simulink model "dimensions_equivalent"  (R2021b)
settings: Solver=VariableStepAuto  StartTime=0.0  StopTime=10.0  RelTol=1e-3
undefined symbols (not defined in the file): DiscIntNeverNeededParam, magnitude, Newton, Raphson
libraries: simulink x80, slpidlib x2
(part 2 of 3)

== system dimensions_equivalent/tsmc_Slforge53 ==
  tsmc_Slforge1 : Inport
  tsmc_Slforge10 : Delay  SampleTime=1
  tsmc_Slforge3 : DiscreteFilter  SampleTime=1
  tsmc_Slforge4 : Sum  Inputs=+-
  tsmc_Slforge5 : Rounding
  tsmc_Slforge6 : ComplexToRealImag
  tsmc_Slforge7 : Product  Inputs=*
  tsmc_Slforge8 : Polyval  Coefs=[ +2.081618890e-019, -1.441693666e-014, +4.719686976e-010, -8.536869453e-006, +1.621573104e-001, -8.087801117e+001 ]
  tsmc_Slforge9 : Delay  SampleTime=1
  tsmc_Slforge2 : Outport  VectorParamsAs1DForOutWhenUnconnected=off
  wires:
  tsmc_Slforge1/1 -> tsmc_Slforge7/1
  tsmc_Slforge7/1 -> tsmc_Slforge3/1
  tsmc_Slforge4/1 -> tsmc_Slforge8/1
  tsmc_Slforge8/1 -> tsmc_Slforge6/1
  tsmc_Slforge6/1 -> tsmc_Slforge5/1
  tsmc_Slforge3/1 -> tsmc_Slforge2/1
  tsmc_Slforge5/1 -> tsmc_Slforge9/1
  tsmc_Slforge9/1 -> tsmc_Slforge4/2
  tsmc_Slforge6/2 -> tsmc_Slforge10/1
  tsmc_Slforge10/1 -> tsmc_Slforge4/1

== system dimensions_equivalent/tsmc_Slforge54 ==
  tsmc_Slforge1 : Inport
  tsmc_Slforge10 : Inport  Port=2
  tsmc_Slforge11 : Inport  Port=3
  tsmc_Slforge3 : Delay  SampleTime=1
  tsmc_Slforge4 : Polyval  Coefs=[ +2.081618890e-019, -1.441693666e-014, +4.719686976e-010, -8.536869453e-006, +1.621573104e-001, -8.087801117e+001 ]
  tsmc_Slforge5 : Sum  Inputs=+-
  tsmc_Slforge6 : Signum
  tsmc_Slforge7 : Product
  tsmc_Slforge8 : Product  Inputs=*
  tsmc_Slforge9 : Constant  Value=[57292007.464946]  SampleTime=1
  tsmc_Slforge2 : Outport  VectorParamsAs1DForOutWhenUnconnected=off
  wires:
  tsmc_Slforge5/1 -> tsmc_Slforge7/1
  tsmc_Slforge9/1 -> tsmc_Slforge4/1
  tsmc_Slforge10/1 -> tsmc_Slforge3/1
  tsmc_Slforge6/1 -> tsmc_Slforge5/1
  tsmc_Slforge3/1 -> tsmc_Slforge2/1
  tsmc_Slforge4/1 -> tsmc_Slforge8/1
  tsmc_Slforge8/1 -> tsmc_Slforge5/2
  tsmc_Slforge1/1 -> tsmc_Slforge7/2
  tsmc_Slforge11/1 -> tsmc_Slforge6/1

== system dimensions_equivalent/tsmc_Slforge55 ==
  tsmc_Slforge1 : Inport
  tsmc_Slforge3 : simulink/Discrete/Transfer Fcn First Order  PoleZ=0.95  ICPrevOutput=0.0  DoSatur=off
  tsmc_Slforge4 : Math  Operator=log10  SignedPower=on  SaturateOnIntegerOverflow=on
  tsmc_Slforge5 : Product
  tsmc_Slforge6 : Product  Inputs=**
  tsmc_Slforge7 : Rounding
  tsmc_Slforge8 : Delay  SampleTime=1
  tsmc_Slforge9 : Delay  SampleTime=1
  tsmc_Slforge2 : Outport  VectorParamsAs1DForOutWhenUnconnected=off
  wires:
  tsmc_Slforge6/1 -> tsmc_Slforge4/1
  tsmc_Slforge7/1 -> tsmc_Slforge2/1, tsmc_Slforge9/1
  tsmc_Slforge1/1 -> tsmc_Slforge6/1
  tsmc_Slforge3/1 -> tsmc_Slforge7/1, tsmc_Slforge5/2
  tsmc_Slforge4/1 -> tsmc_Slforge5/1
  tsmc_Slforge5/1 -> tsmc_Slforge8/1
  tsmc_Slforge8/1 -> tsmc_Slforge6/2
  tsmc_Slforge9/1 -> tsmc_Slforge3/1

== system dimensions_equivalent/tsmc_Slforge56 ==
  tsmc_Slforge1 : Inport
  tsmc_Slforge10 : Delay  SampleTime=1
  tsmc_Slforge3 : DiscreteFir  SampleTime=1
  tsmc_Slforge4 : Rounding
  tsmc_Slforge5 : Reshape
  tsmc_Slforge6 : Bias  Bias=[938444470.111902]
  tsmc_Slforge7 : Squeeze
  tsmc_Slforge8 : Trigonometry
  tsmc_Slforge9 : Delay  SampleTime=1
  tsmc_Slforge2 : Outport  VectorParamsAs1DForOutWhenUnconnected=off
  wires:
  tsmc_Slforge4/1 -> tsmc_Slforge6/1
  tsmc_Slforge6/1 -> tsmc_Slforge2/1
  tsmc_Slforge5/1 -> tsmc_Slforge7/1
  tsmc_Slforge3/1 -> tsmc_Slforge8/1
  tsmc_Slforge1/1 -> tsmc_Slforge4/1
  tsmc_Slforge8/1 -> tsmc_Slforge9/1
  tsmc_Slforge9/1 -> tsmc_Slforge3/1
  tsmc_Slforge7/1 -> tsmc_Slforge10/1
  tsmc_Slforge10/1 -> tsmc_Slforge5/1

== system dimensions_equivalent/tsmc_Slforge74 ==
  tsmc_Slforge1 : Inport
  tsmc_Slforge23 : Inport  Port=2
  tsmc_Slforge24 : Inport  Port=3
  tsmc_Slforge25 : Inport  Port=4
  Action Port : ActionPort  ActionPortLabel=if { }
  tsmc_Slforge10 : MinMax  Function=max  Inputs=2
  tsmc_Slforge11 : Gain  Gain=[-950435742.515709]
  tsmc_Slforge12 : Sin  TimeSource=Use external signal  SampleTime=0
  tsmc_Slforge13 : Product  Inputs=*
  tsmc_Slforge14 : MinMax  Inputs=3
  tsmc_Slforge15 : Squeeze
  tsmc_Slforge16 : Sum  Inputs=+
  tsmc_Slforge17 : Polyval  Coefs=[ +2.081618890e-019, -1.441693666e-014, +4.719686976e-010, -8.536869453e-006, +1.621573104e-001, -8.087801117e+001 ]
  tsmc_Slforge18 : DotProduct  InputSameDT=on  OutDataTypeStr=Inherit: Inherit via internal rule
  tsmc_Slforge19 : Sin  TimeSource=Use external signal  SampleTime=0
  tsmc_Slforge20 : Sum  Inputs=-+
  tsmc_Slforge21 : Constant  Value=[772260001.144114]  SampleTime=1
  tsmc_Slforge22 : Constant  Value=[-948406195.487638]  SampleTime=1
  tsmc_Slforge26 : Delay
  tsmc_Slforge27 : Delay
  tsmc_Slforge3 : simulink/Discrete/Transfer Fcn Real Zero  ZeroZ=0.75  ICPrevInput=0.0  DoSatur=off
      settings: SourceProductBaseCode=SL
  tsmc_Slforge4 : simulink/Discrete/Transfer Fcn Lead or Lag  PoleZ=0.95  ZeroZ=0.75  ICPrevOutput=0.0  ICPrevInput=0.0  DoSatur=off
      settings: SourceProductBaseCode=SL
  tsmc_Slforge5 : Sum  Inputs=+-
  tsmc_Slforge6 : simulink/Math Operations/Slider Gain  gain=1  low=0  high=2
  tsmc_Slforge7 : Sqrt  Operator=rSqrt  AlgorithmType=Newton-Raphson  SaturateOnIntegerOverflow=on
  tsmc_Slforge8 : Product
  tsmc_Slforge9 : Sum
  tsmc_Slforge2 : Outport  VectorParamsAs1DForOutWhenUnconnected=off
  wires:
  tsmc_Slforge16/1 -> tsmc_Slforge15/1
  tsmc_Slforge23/1 -> tsmc_Slforge3/1, tsmc_Slforge19/1
  tsmc_Slforge25/1 -> tsmc_Slforge17/1
  tsmc_Slforge21/1 -> tsmc_Slforge20/1
  tsmc_Slforge4/1 -> tsmc_Slforge7/1
  tsmc_Slforge20/1 -> tsmc_Slforge2/1
  tsmc_Slforge6/1 -> tsmc_Slforge18/1
  tsmc_Slforge3/1 -> tsmc_Slforge5/2
  tsmc_Slforge18/1 -> tsmc_Slforge9/1
  tsmc_Slforge17/1 -> tsmc_Slforge10/1
  tsmc_Slforge12/1 -> tsmc_Slforge11/1
  tsmc_Slforge13/1 -> tsmc_Slforge8/1
  tsmc_Slforge8/1 -> tsmc_Slforge20/2
  tsmc_Slforge14/1 -> tsmc_Slforge6/1
  tsmc_Slforge22/1 -> tsmc_Slforge18/2, tsmc_Slforge4/1
  tsmc_Slforge24/1 -> tsmc_Slforge13/1
  tsmc_Slforge9/1 -> tsmc_Slforge10/2
  tsmc_Slforge15/1 -> tsmc_Slforge14/2
  tsmc_Slforge1/1 -> tsmc_Slforge8/2
  tsmc_Slforge5/1 -> tsmc_Slforge12/1
  tsmc_Slforge19/1 -> tsmc_Slforge16/1, tsmc_Slforge9/2
  tsmc_Slforge7/1 -> tsmc_Slforge14/3
  tsmc_Slforge11/1 -> tsmc_Slforge26/1
  tsmc_Slforge26/1 -> tsmc_Slforge5/1
  tsmc_Slforge10/1 -> tsmc_Slforge27/1
  tsmc_Slforge27/1 -> tsmc_Slforge14/1

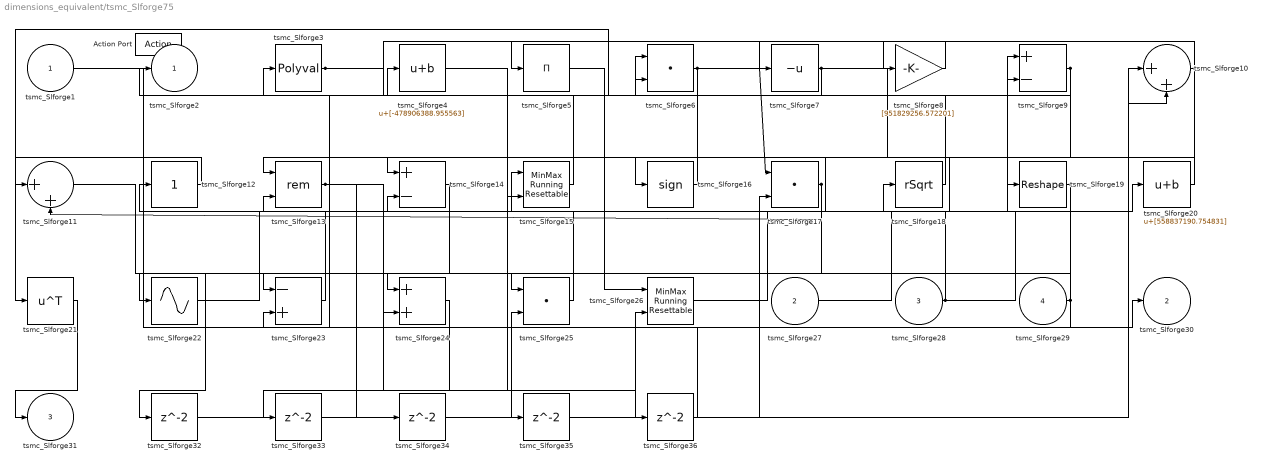
== system dimensions_equivalent/tsmc_Slforge75 ==
  tsmc_Slforge1 : Inport
  tsmc_Slforge27 : Inport  Port=2
  tsmc_Slforge28 : Inport  Port=3
  tsmc_Slforge29 : Inport  Port=4
  Action Port : ActionPort  ActionPortLabel=else { }
  tsmc_Slforge10 : Sum  Inputs=|++
  tsmc_Slforge11 : Sum  Inputs=|++
  tsmc_Slforge12 : simulink/Math Operations/Slider Gain  gain=1  low=0  high=2
  tsmc_Slforge13 : Math  Operator=rem  SignedPower=on  SaturateOnIntegerOverflow=on
  tsmc_Slforge14 : Sum  Inputs=+-
  tsmc_Slforge15 : simulink/Math Operations/MinMax Running Resettable  Function=min  vinit=0.0
  tsmc_Slforge16 : Signum
  tsmc_Slforge17 : DotProduct  InputSameDT=on  OutDataTypeStr=Inherit: Inherit via internal rule
  tsmc_Slforge18 : Sqrt  Operator=rSqrt  AlgorithmType=Newton-Raphson  SaturateOnIntegerOverflow=on
  tsmc_Slforge19 : Reshape
  tsmc_Slforge20 : Bias  Bias=[558837190.754831]
  tsmc_Slforge21 : Math  Operator=transpose  SignedPower=on  SaturateOnIntegerOverflow=on
  tsmc_Slforge22 : Sin  TimeSource=Use external signal  SampleTime=0
  tsmc_Slforge23 : Sum  Inputs=-+
  tsmc_Slforge24 : Sum
  tsmc_Slforge25 : DotProduct  InputSameDT=on  OutDataTypeStr=Inherit: Inherit via internal rule
  tsmc_Slforge26 : simulink/Math Operations/MinMax Running Resettable  Function=min  vinit=0.0
  tsmc_Slforge3 : Polyval  Coefs=[ +2.081618890e-019, -1.441693666e-014, +4.719686976e-010, -8.536869453e-006, +1.621573104e-001, -8.087801117e+001 ]
  tsmc_Slforge{32..36} (5 alike) : Delay
  tsmc_Slforge4 : Bias  Bias=[-478906388.955563]
  tsmc_Slforge5 : Product  Inputs=*
  tsmc_Slforge6 : DotProduct  InputSameDT=on  OutDataTypeStr=Inherit: Inherit via internal rule
  tsmc_Slforge7 : UnaryMinus
  tsmc_Slforge8 : Gain  Gain=[951829256.572201]
  tsmc_Slforge9 : Sum  Inputs=+-
  tsmc_Slforge2 : Outport  VectorParamsAs1DForOutWhenUnconnected=off
  tsmc_Slforge30 : Outport  Port=2  VectorParamsAs1DForOutWhenUnconnected=off
  tsmc_Slforge31 : Outport  Port=3  VectorParamsAs1DForOutWhenUnconnected=off
  wires:
  tsmc_Slforge28/1 -> tsmc_Slforge20/1, tsmc_Slforge15/1
  tsmc_Slforge1/1 -> tsmc_Slforge30/1
  tsmc_Slforge5/1 -> tsmc_Slforge26/1
  tsmc_Slforge18/1 -> tsmc_Slforge21/1
  tsmc_Slforge17/1 -> tsmc_Slforge25/1, tsmc_Slforge11/2
  tsmc_Slforge9/1 -> tsmc_Slforge16/1, tsmc_Slforge2/1
  tsmc_Slforge15/1 -> tsmc_Slforge4/1
  tsmc_Slforge19/1 -> tsmc_Slforge24/1, tsmc_Slforge24/2
  tsmc_Slforge25/1 -> tsmc_Slforge12/1
  tsmc_Slforge11/1 -> tsmc_Slforge23/1
  tsmc_Slforge10/1 -> tsmc_Slforge14/1, tsmc_Slforge7/1
  tsmc_Slforge8/1 -> tsmc_Slforge5/1
  tsmc_Slforge16/1 -> tsmc_Slforge6/1
  tsmc_Slforge21/1 -> tsmc_Slforge31/1
  tsmc_Slforge29/1 -> tsmc_Slforge18/1, tsmc_Slforge22/1, tsmc_Slforge23/2
  tsmc_Slforge22/1 -> tsmc_Slforge14/2
  tsmc_Slforge12/1 -> tsmc_Slforge11/1
  tsmc_Slforge20/1 -> tsmc_Slforge13/1
  tsmc_Slforge6/1 -> tsmc_Slforge17/1, tsmc_Slforge15/2
  tsmc_Slforge23/1 -> tsmc_Slforge13/2
  tsmc_Slforge26/1 -> tsmc_Slforge10/2
  tsmc_Slforge27/1 -> tsmc_Slforge9/1
  tsmc_Slforge7/1 -> tsmc_Slforge19/1, tsmc_Slforge6/2
  tsmc_Slforge3/1 -> tsmc_Slforge8/1, tsmc_Slforge9/2
  tsmc_Slforge13/1 -> tsmc_Slforge34/1, tsmc_Slforge35/1
  tsmc_Slforge14/1 -> tsmc_Slforge32/1
  tsmc_Slforge32/1 -> tsmc_Slforge26/2
  tsmc_Slforge24/1 -> tsmc_Slforge33/1
  tsmc_Slforge33/1 -> tsmc_Slforge10/1
  tsmc_Slforge34/1 -> tsmc_Slforge25/2
  tsmc_Slforge35/1 -> tsmc_Slforge17/2
  tsmc_Slforge4/1 -> tsmc_Slforge36/1
  tsmc_Slforge36/1 -> tsmc_Slforge3/1

== system dimensions_equivalent/tsmc_Slforge76 ==
  tsmc_Slforge1 : Inport
  tsmc_Slforge23 : Inport  Port=2
  Action Port : ActionPort  ActionPortLabel=if { }
  tsmc_Slforge10 : PermuteDimensions
  tsmc_Slforge11 : simulink/Math Operations/Slider Gain  gain=1  low=0  high=2
  tsmc_Slforge12 : Product  Inputs=*
  tsmc_Slforge13 : Assignment  DiagnosticForDimensions=Warning  IndexOptions=Index vector (dialog)  Indices=1  OutputSizes=1
  tsmc_Slforge14 : Sum  Inputs=+-
  tsmc_Slforge15 : Sqrt  SaturateOnIntegerOverflow=on
  tsmc_Slforge16 : MinMax  Function=max  Inputs=3
  tsmc_Slforge17 : Trigonometry
  tsmc_Slforge18 : simulink/Math Operations/Slider Gain  gain=1  low=0  high=2
  tsmc_Slforge19 : Sum  Inputs=+
  tsmc_Slforge20 : Bias  Bias=[872641712.418496]
  tsmc_Slforge21 : Constant  Value=[-855607815.894000]  SampleTime=1
  tsmc_Slforge22 : Constant  Value=[-549961710.513613]  SampleTime=1
  tsmc_Slforge{3,25..28} (5 alike) : Delay
  tsmc_Slforge4 : simulink/Discrete/Tapped Delay  vinit=0.0  samptime=-1  NumDelays=1  DelayOrder=Oldest  includeCurrent=off
  tsmc_Slforge5 : Delay  DelayLengthSource=Input port
      settings: InputPortMap=u0,p1
  tsmc_Slforge6 : Sum  Inputs=--
  tsmc_Slforge7 : Sqrt  SaturateOnIntegerOverflow=on
  tsmc_Slforge8 : Sum  Inputs=--
  tsmc_Slforge9 : Sin  TimeSource=Use external signal  SampleTime=0
  tsmc_Slforge2 : Outport  VectorParamsAs1DForOutWhenUnconnected=off
  tsmc_Slforge24 : Outport  Port=2  VectorParamsAs1DForOutWhenUnconnected=off
  wires:
  tsmc_Slforge8/1 -> tsmc_Slforge16/1, tsmc_Slforge13/2
  tsmc_Slforge4/1 -> tsmc_Slforge5/1
  tsmc_Slforge12/1 -> tsmc_Slforge6/1
  tsmc_Slforge6/1 -> tsmc_Slforge10/1
  tsmc_Slforge5/1 -> tsmc_Slforge18/1
  tsmc_Slforge14/1 -> tsmc_Slforge9/1
  tsmc_Slforge22/1 -> tsmc_Slforge13/1
  tsmc_Slforge18/1 -> tsmc_Slforge11/1, tsmc_Slforge2/1
  tsmc_Slforge3/1 -> tsmc_Slforge15/1
  tsmc_Slforge16/1 -> tsmc_Slforge24/1
  tsmc_Slforge19/1 -> tsmc_Slforge12/1
  tsmc_Slforge13/1 -> tsmc_Slforge17/1
  tsmc_Slforge9/1 -> tsmc_Slforge8/1, tsmc_Slforge16/3
  tsmc_Slforge21/1 -> tsmc_Slforge19/1
  tsmc_Slforge10/1 -> tsmc_Slforge7/1, tsmc_Slforge20/1, tsmc_Slforge8/2
  tsmc_Slforge1/1 -> tsmc_Slforge14/2
  tsmc_Slforge11/1 -> tsmc_Slforge6/2
  tsmc_Slforge23/1 -> tsmc_Slforge16/2
  tsmc_Slforge17/1 -> tsmc_Slforge25/1
  tsmc_Slforge25/1 -> tsmc_Slforge14/1
  tsmc_Slforge15/1 -> tsmc_Slforge26/1
  tsmc_Slforge26/1 -> tsmc_Slforge3/1
  tsmc_Slforge7/1 -> tsmc_Slforge27/1
  tsmc_Slforge27/1 -> tsmc_Slforge4/1
  tsmc_Slforge20/1 -> tsmc_Slforge28/1
  tsmc_Slforge28/1 -> tsmc_Slforge5/2

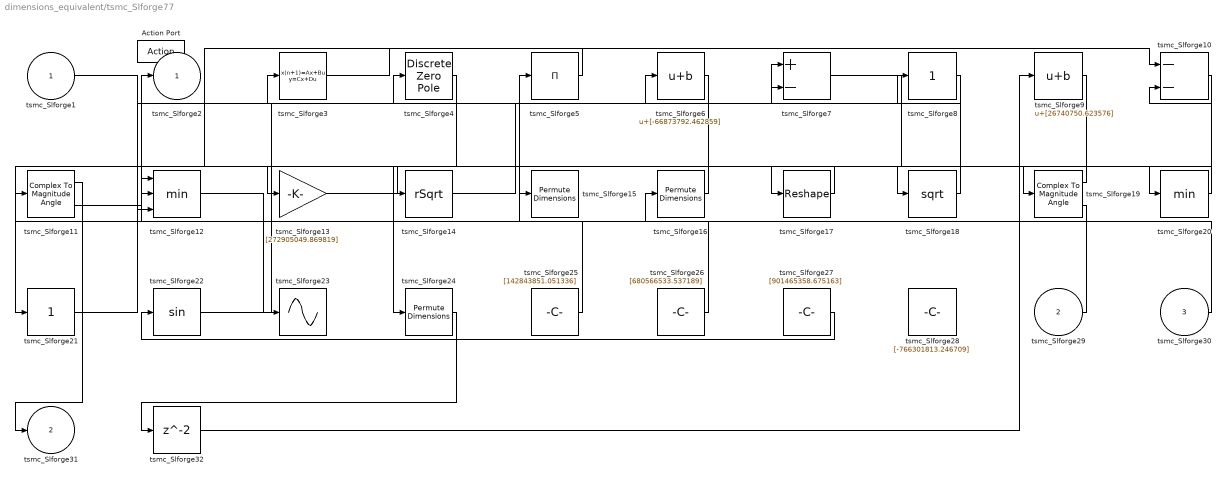
== system dimensions_equivalent/tsmc_Slforge77 ==
  tsmc_Slforge1 : Inport
  tsmc_Slforge29 : Inport  Port=2
  tsmc_Slforge30 : Inport  Port=3
  Action Port : ActionPort  ActionPortLabel=else { }
  tsmc_Slforge10 : Sum  Inputs=--
  tsmc_Slforge11 : ComplexToMagnitudeAngle
  tsmc_Slforge12 : MinMax  Inputs=3
  tsmc_Slforge13 : Gain  Gain=[272905049.869819]
  tsmc_Slforge14 : Sqrt  Operator=rSqrt  AlgorithmType=Newton-Raphson  SaturateOnIntegerOverflow=on
  tsmc_Slforge15 : PermuteDimensions
  tsmc_Slforge16 : PermuteDimensions
  tsmc_Slforge17 : Reshape
  tsmc_Slforge18 : Sqrt  SaturateOnIntegerOverflow=on
  tsmc_Slforge19 : ComplexToMagnitudeAngle
  tsmc_Slforge20 : MinMax
  tsmc_Slforge21 : simulink/Math Operations/Slider Gain  gain=1  low=0  high=2
  tsmc_Slforge22 : Trigonometry
  tsmc_Slforge23 : Sin  TimeSource=Use external signal  SampleTime=0
  tsmc_Slforge24 : PermuteDimensions
  tsmc_Slforge25 : Constant  Value=[142843851.051336]  SampleTime=1
  tsmc_Slforge26 : Constant  Value=[680566533.537189]  SampleTime=1
  tsmc_Slforge27 : Constant  Value=[901465358.675163]  SampleTime=1
  tsmc_Slforge28 : Constant  Value=[-766301813.246709]  SampleTime=1
  tsmc_Slforge3 : DiscreteStateSpace  SampleTime=-1
  tsmc_Slforge32 : Delay
  tsmc_Slforge4 : DiscreteZeroPole  Poles=[0 0.5]  Gain=1  SampleTime=-1
  tsmc_Slforge5 : Product  Inputs=*
  tsmc_Slforge6 : Bias  Bias=[-66873792.462859]
  tsmc_Slforge7 : Sum  Inputs=+-
  tsmc_Slforge8 : simulink/Math Operations/Slider Gain  gain=1  low=0  high=2
  tsmc_Slforge9 : Bias  Bias=[26740750.623576]
  tsmc_Slforge2 : Outport  VectorParamsAs1DForOutWhenUnconnected=off
  tsmc_Slforge31 : Outport  Port=2  VectorParamsAs1DForOutWhenUnconnected=off
  wires:
  tsmc_Slforge30/1 -> tsmc_Slforge5/1
  tsmc_Slforge5/1 -> tsmc_Slforge21/1
  tsmc_Slforge22/1 -> tsmc_Slforge4/1
  tsmc_Slforge13/1 -> tsmc_Slforge20/1
  tsmc_Slforge17/1 -> tsmc_Slforge15/1
  tsmc_Slforge9/1 -> tsmc_Slforge24/1
  tsmc_Slforge27/1 -> tsmc_Slforge22/1
  tsmc_Slforge18/1 -> tsmc_Slforge7/1
  tsmc_Slforge4/1 -> tsmc_Slforge13/1
  tsmc_Slforge25/1 -> tsmc_Slforge11/1
  tsmc_Slforge14/1 -> tsmc_Slforge7/2
  tsmc_Slforge16/1 -> tsmc_Slforge6/1
  tsmc_Slforge21/1 -> tsmc_Slforge3/1
  tsmc_Slforge8/1 -> tsmc_Slforge18/1
  tsmc_Slforge3/1 -> tsmc_Slforge10/1
  tsmc_Slforge29/1 -> tsmc_Slforge14/1
  tsmc_Slforge26/1 -> tsmc_Slforge2/1
  tsmc_Slforge19/1 -> tsmc_Slforge17/1
  tsmc_Slforge20/1 -> tsmc_Slforge10/2
  tsmc_Slforge6/1 -> tsmc_Slforge12/1
  tsmc_Slforge11/1 -> tsmc_Slforge31/1
  tsmc_Slforge19/2 -> tsmc_Slforge16/1
  tsmc_Slforge12/1 -> tsmc_Slforge23/1
  tsmc_Slforge11/2 -> tsmc_Slforge12/2
  tsmc_Slforge7/1 -> tsmc_Slforge19/1
  tsmc_Slforge1/1 -> tsmc_Slforge8/1
  tsmc_Slforge10/1 -> tsmc_Slforge12/3
  tsmc_Slforge24/1 -> tsmc_Slforge32/1
  tsmc_Slforge32/1 -> tsmc_Slforge9/1

== system dimensions_equivalent/tsmc_Slforge78 ==
  tsmc_Slforge1 : Inport
  tsmc_Slforge20 : Inport  Port=2
  tsmc_Slforge21 : Inport  Port=3
  tsmc_Slforge22 : Inport  Port=4
  tsmc_Slforge23 : Inport  Port=5
  tsmc_Slforge24 : Inport  Port=6
  Action Port : ActionPort  ActionPortLabel=if { }
  tsmc_Slforge10 : MinMax  Function=max  Inputs=2
  tsmc_Slforge11 : Reshape
  tsmc_Slforge12 : Bias  Bias=[772438842.352747]
  tsmc_Slforge13 : Polyval  Coefs=[ +2.081618890e-019, -1.441693666e-014, +4.719686976e-010, -8.536869453e-006, +1.621573104e-001, -8.087801117e+001 ]
  tsmc_Slforge14 : Squeeze
  tsmc_Slforge15 : MinMax  Function=max
  tsmc_Slforge16 : MinMax  Function=max  Inputs=3
  tsmc_Slforge17 : Constant  Value=[-48406649.687781]  SampleTime=1
  tsmc_Slforge18 : Constant  Value=[-479832900.428704]  SampleTime=1
  tsmc_Slforge19 : Constant  Value=[314816186.317253]  SampleTime=1
  tsmc_Slforge3 : simulink/Discrete/Difference  ICPrevInput=0.0  OutMin=[]  OutMax=[]  OutDataTypeStr=Inherit: Inherit via back propagation  OutDataType=fixdt(1, 16)  OutScaling=2^-10  DoSatur=off
  tsmc_Slforge4 : simulink/Continuous/PID Controller (2DOF)  Controller=PID  TimeDomain=Discrete-time  SampleTime=-1  IntegratorMethod=Forward Euler  FilterMethod=Forward Euler  Form=Parallel  UseFilter=on  ControllerParametersSource=internal  P=1  I=1  D=0  N=100  b=1  c=1  InitialConditionSource=internal  InitialConditionForIntegrator=0  InitialConditionForFilter=0  ExternalReset=none  LimitOutput=off  UpperSaturationLimit=inf  LowerSaturationLimit=-inf  LinearizeAsGain=off  AntiWindupMode=none  Kb=1  TrackingMode=off  Kt=1  PParamMin=[]  PParamMax=[]  IParamMin=[]  IParamMax=[]  DParamMin=[]  DParamMax=[]  NParamMin=[]  NParamMax=[]  bParamMin=[]  bParamMax=[]  cParamMin=[]  cParamMax=[]  KbParamMin=[]  KbParamMax=[]  KtParamMin=[]  KtParamMax=[]  POutMin=[]  POutMax=[]  IOutMin=[]  IOutMax=[]  DOutMin=[]  DOutMax=[]  NOutMin=[]  NOutMax=[]  bOutMin=[]  bOutMax=[]  cOutMin=[]  cOutMax=[]  KbOutMin=[]  KbOutMax=[]  KtOutMin=[]  KtOutMax=[]  IntegratorOutMin=[]  IntegratorOutMax=[]  FilterOutMin=[]  FilterOutMax=[]  SumOutMin=[]  SumOutMax=[]  Sum1OutMin=[]  Sum1OutMax=[]  Sum2OutMin=[]  Sum2OutMax=[]  Sum3OutMin=[]  Sum3OutMax=[]  SumI1OutMin=[]  SumI1OutMax=[]  SumI2OutMin=[]  SumI2OutMax=[]  SumI3OutMin=[]  SumI3OutMax=[]  SumDOutMin=[]  SumDOutMax=[]  SaturationOutMin=[]  SaturationOutMax=[]  IntegratorContinuousStateAttributes=''  IntegratorStateMustResolveToSignalObject=off  IntegratorRTWStateStorageClass=Auto  FilterContinuousStateAttributes=''  FilterStateMustResolveToSignalObject=off  FilterRTWStateStorageClass=Auto  DifferentiatorICPrevScaledInput=0  DifferentiatorOutMin=[]  DifferentiatorOutMax=[]  FilterDiffOutCoefMin=[]  FilterDiffOutCoefMax=[]  SumDenOutMin=[]  SumDenOutMax=[]  SumNumOutMin=[]  SumNumOutMax=[]  ReciprocalOutMin=[]  ReciprocalOutMax=[]  DivideOutMin=[]  DivideOutMax=[]  TunerSelectOption=Transfer Function Based (PID Tuner App)
  tsmc_Slforge5 : Polyval  Coefs=[ +2.081618890e-019, -1.441693666e-014, +4.719686976e-010, -8.536869453e-006, +1.621573104e-001, -8.087801117e+001 ]
  tsmc_Slforge6 : Sqrt  Operator=rSqrt  AlgorithmType=Newton-Raphson  SaturateOnIntegerOverflow=on
  tsmc_Slforge7 : Sqrt  Operator=rSqrt  AlgorithmType=Newton-Raphson  SaturateOnIntegerOverflow=on
  tsmc_Slforge8 : simulink/Math Operations/MinMax Running Resettable  Function=min  vinit=0.0
  tsmc_Slforge9 : Rounding
  tsmc_Slforge2 : Outport  VectorParamsAs1DForOutWhenUnconnected=off
  wires:
  tsmc_Slforge13/1 -> tsmc_Slforge5/1
  tsmc_Slforge6/1 -> tsmc_Slforge8/1
  tsmc_Slforge14/1 -> tsmc_Slforge8/2
  tsmc_Slforge11/1 -> tsmc_Slforge3/1
  tsmc_Slforge20/1 -> tsmc_Slforge12/1
  tsmc_Slforge17/1 -> tsmc_Slforge6/1
  tsmc_Slforge22/1 -> tsmc_Slforge2/1
  tsmc_Slforge24/1 -> tsmc_Slforge16/1
  tsmc_Slforge12/1 -> tsmc_Slforge11/1
  tsmc_Slforge3/1 -> tsmc_Slforge15/1
  tsmc_Slforge7/1 -> tsmc_Slforge4/1
  tsmc_Slforge4/1 -> tsmc_Slforge13/1
  tsmc_Slforge8/1 -> tsmc_Slforge7/1
  tsmc_Slforge10/1 -> tsmc_Slforge14/1
  tsmc_Slforge21/1 -> tsmc_Slforge16/2
  tsmc_Slforge1/1 -> tsmc_Slforge9/1
  tsmc_Slforge23/1 -> tsmc_Slforge10/1
  tsmc_Slforge18/1 -> tsmc_Slforge4/2
  tsmc_Slforge15/1 -> tsmc_Slforge10/2
  tsmc_Slforge19/1 -> tsmc_Slforge16/3

== system dimensions_equivalent/tsmc_Slforge79 ==
  tsmc_Slforge1 : Inport
  Action Port : ActionPort  ActionPortLabel=else { }
  tsmc_Slforge10 : UnaryMinus
  tsmc_Slforge11 : Sqrt  Operator=rSqrt  AlgorithmType=Newton-Raphson  SaturateOnIntegerOverflow=on
  tsmc_Slforge12 : Product  Inputs=*
  tsmc_Slforge13 : Abs
  tsmc_Slforge14 : Sum  Inputs=+
  tsmc_Slforge15 : Sum  Inputs=+-
  tsmc_Slforge16 : Squeeze
  tsmc_Slforge17 : Signum
  tsmc_Slforge18 : Sum  Inputs=+-
  tsmc_Slforge19 : Product  Inputs=**
  tsmc_Slforge20 : Math  SignedPower=on  SaturateOnIntegerOverflow=on
  tsmc_Slforge21 : Constant  Value=[678233117.129764]  SampleTime=1
  tsmc_Slforge22 : Constant  Value=[-306944065.535399]  SampleTime=1
  tsmc_Slforge23 : Delay
  tsmc_Slforge3 : Delay  ShowEnablePort=on
      settings: InputPortMap=u0,e6
  tsmc_Slforge4 : simulink/Discrete/Tapped Delay  vinit=0.0  samptime=-1  NumDelays=1  DelayOrder=Oldest  includeCurrent=off
  tsmc_Slforge5 : simulink/Discrete/Difference  ICPrevInput=0.0  OutMin=[]  OutMax=[]  OutDataTypeStr=Inherit: Inherit via back propagation  OutDataType=fixdt(1, 16)  OutScaling=2^-10  DoSatur=off
  tsmc_Slforge6 : simulink/Discrete/Difference  ICPrevInput=0.0  OutMin=[]  OutMax=[]  OutDataTypeStr=Inherit: Inherit via back propagation  OutDataType=fixdt(1, 16)  OutScaling=2^-10  DoSatur=off
  tsmc_Slforge7 : simulink/Math Operations/MinMax Running Resettable  Function=min  vinit=0.0
  tsmc_Slforge8 : MinMax  Inputs=2
  tsmc_Slforge9 : PermuteDimensions
  tsmc_Slforge2 : Outport  VectorParamsAs1DForOutWhenUnconnected=off
  wires:
  tsmc_Slforge11/1 -> tsmc_Slforge7/1
  tsmc_Slforge9/1 -> tsmc_Slforge6/1
  tsmc_Slforge10/1 -> tsmc_Slforge19/1
  tsmc_Slforge18/1 -> tsmc_Slforge3/2
  tsmc_Slforge6/1 -> tsmc_Slforge12/1
  tsmc_Slforge1/1 -> tsmc_Slforge19/2
  tsmc_Slforge7/1 -> tsmc_Slforge8/1
  tsmc_Slforge5/1 -> tsmc_Slforge4/1
  tsmc_Slforge19/1 -> tsmc_Slforge15/1, tsmc_Slforge15/2
  tsmc_Slforge14/1 -> tsmc_Slforge7/2, tsmc_Slforge13/1
  tsmc_Slforge20/1 -> tsmc_Slforge18/1
  tsmc_Slforge22/1 -> tsmc_Slforge10/1, tsmc_Slforge14/1, tsmc_Slforge18/2
  tsmc_Slforge21/1 -> tsmc_Slforge17/1
  tsmc_Slforge17/1 -> tsmc_Slforge9/1
  tsmc_Slforge12/1 -> tsmc_Slforge8/2
  tsmc_Slforge13/1 -> tsmc_Slforge20/1
  tsmc_Slforge3/1 -> tsmc_Slforge5/1
  tsmc_Slforge4/1 -> tsmc_Slforge16/1
  tsmc_Slforge8/1 -> tsmc_Slforge2/1
  tsmc_Slforge15/1 -> tsmc_Slforge11/1
  tsmc_Slforge16/1 -> tsmc_Slforge23/1
  tsmc_Slforge23/1 -> tsmc_Slforge3/1

== system dimensions_equivalent/tsmc_Slforge80 ==
  tsmc_Slforge1 : Inport
  tsmc_Slforge21 : Inport  Port=2
  Action Port : ActionPort  ActionPortLabel=if { }
  tsmc_Slforge10 : Squeeze
  tsmc_Slforge11 : Sqrt  SaturateOnIntegerOverflow=on
  tsmc_Slforge12 : Reshape
  tsmc_Slforge13 : Gain  Gain=[-764094660.607144]
  tsmc_Slforge14 : Squeeze
  tsmc_Slforge15 : Sum  Inputs=|++
  tsmc_Slforge16 : Abs
  tsmc_Slforge17 : Sum  Inputs=+
  tsmc_Slforge18 : PermuteDimensions
  tsmc_Slforge19 : Sum  Inputs=|++
  tsmc_Slforge20 : Constant  Value=[275262453.457790]  SampleTime=1
  tsmc_Slforge23 : Delay
  tsmc_Slforge24 : Delay
  tsmc_Slforge3 : simulink/Discrete/Transfer Fcn Lead or Lag  PoleZ=0.95  ZeroZ=0.75  ICPrevOutput=0.0  ICPrevInput=0.0  DoSatur=off
      settings: SourceProductBaseCode=SL
  tsmc_Slforge4 : DiscreteStateSpace  SampleTime=-1
  tsmc_Slforge5 : Delay  DelayLengthSource=Input port
      settings: InputPortMap=u0,p1
  tsmc_Slforge6 : Delay  DelayLengthSource=Input port
      settings: InputPortMap=u0,p1
  tsmc_Slforge7 : simulink/Math Operations/Slider Gain  gain=1  low=0  high=2
  tsmc_Slforge8 : ComplexToMagnitudeAngle
  tsmc_Slforge9 : Sum  Inputs=+-
  tsmc_Slforge2 : Outport  VectorParamsAs1DForOutWhenUnconnected=off
  tsmc_Slforge22 : Outport  Port=2  VectorParamsAs1DForOutWhenUnconnected=off
  wires:
  tsmc_Slforge4/1 -> tsmc_Slforge15/1
  tsmc_Slforge13/1 -> tsmc_Slforge9/1
  tsmc_Slforge8/1 -> tsmc_Slforge7/1
  tsmc_Slforge17/1 -> tsmc_Slforge13/1, tsmc_Slforge19/2
  tsmc_Slforge3/1 -> tsmc_Slforge18/1
  tsmc_Slforge16/1 -> tsmc_Slforge22/1, tsmc_Slforge11/1
  tsmc_Slforge12/1 -> tsmc_Slforge8/1
  tsmc_Slforge8/2 -> tsmc_Slforge4/1, tsmc_Slforge24/1
  tsmc_Slforge7/1 -> tsmc_Slforge14/1
  tsmc_Slforge1/1 -> tsmc_Slforge17/1
  tsmc_Slforge20/1 -> tsmc_Slforge9/2
  tsmc_Slforge9/1 -> tsmc_Slforge5/1
  tsmc_Slforge18/1 -> tsmc_Slforge12/1
  tsmc_Slforge19/1 -> tsmc_Slforge3/1
  tsmc_Slforge14/1 -> tsmc_Slforge2/1
  tsmc_Slforge11/1 -> tsmc_Slforge15/2
  tsmc_Slforge21/1 -> tsmc_Slforge6/1
  tsmc_Slforge5/1 -> tsmc_Slforge6/2
  tsmc_Slforge6/1 -> tsmc_Slforge10/1
  tsmc_Slforge10/1 -> tsmc_Slforge16/1
  tsmc_Slforge15/1 -> tsmc_Slforge23/1
  tsmc_Slforge23/1 -> tsmc_Slforge5/2
  tsmc_Slforge24/1 -> tsmc_Slforge19/1

== system dimensions_equivalent/tsmc_Slforge81 ==
  tsmc_Slforge1 : Inport
  tsmc_Slforge24 : Inport  Port=2
  tsmc_Slforge25 : Inport  Port=3
  Action Port : ActionPort  ActionPortLabel=else { }
  tsmc_Slforge10 : Bias  Bias=[-344768732.207249]
  tsmc_Slforge11 : simulink/Math Operations/Slider Gain  gain=1  low=0  high=2
  tsmc_Slforge12 : PermuteDimensions
  tsmc_Slforge13 : simulink/Math Operations/Slider Gain  gain=1  low=0  high=2
  tsmc_Slforge14 : Sum  Inputs=+-
  tsmc_Slforge15 : Bias  Bias=[-933685166.648832]
  tsmc_Slforge16 : Sqrt  SaturateOnIntegerOverflow=on
  tsmc_Slforge17 : Assignment  DiagnosticForDimensions=Warning  IndexOptions=Index vector (dialog)  Indices=1  OutputSizes=1
  tsmc_Slforge18 : Squeeze
  tsmc_Slforge19 : Rounding
  tsmc_Slforge20 : Math  Operator=pow  SignedPower=on  SaturateOnIntegerOverflow=on
  tsmc_Slforge21 : Sum  Inputs=-+
  tsmc_Slforge22 : simulink/Math Operations/MinMax Running Resettable  Function=min  vinit=0.0
  tsmc_Slforge23 : Constant  Value=[662195432.123307]  SampleTime=1
  tsmc_Slforge26 : Delay
  tsmc_Slforge27 : Delay
  tsmc_Slforge3 : simulink/Discrete/Transfer Fcn Lead or Lag  PoleZ=0.95  ZeroZ=0.75  ICPrevOutput=0.0  ICPrevInput=0.0  DoSatur=off
      settings: SourceProductBaseCode=SL
  tsmc_Slforge4 : simulink/Discrete/Transfer Fcn First Order  PoleZ=0.95  ICPrevOutput=0.0  DoSatur=off
  tsmc_Slforge5 : DotProduct  InputSameDT=on  OutDataTypeStr=Inherit: Inherit via internal rule
  tsmc_Slforge6 : Rounding
  tsmc_Slforge7 : Reshape
  tsmc_Slforge8 : ComplexToMagnitudeAngle
  tsmc_Slforge9 : Bias  Bias=[902734951.405075]
  tsmc_Slforge2 : Outport  VectorParamsAs1DForOutWhenUnconnected=off
  wires:
  tsmc_Slforge20/1 -> tsmc_Slforge7/1
  tsmc_Slforge11/1 -> tsmc_Slforge8/1
  tsmc_Slforge15/1 -> tsmc_Slforge11/1
  tsmc_Slforge21/1 -> tsmc_Slforge2/1
  tsmc_Slforge8/1 -> tsmc_Slforge9/1
  tsmc_Slforge5/1 -> tsmc_Slforge17/1
  tsmc_Slforge24/1 -> tsmc_Slforge12/1
  tsmc_Slforge13/1 -> tsmc_Slforge19/1
  tsmc_Slforge23/1 -> tsmc_Slforge10/1
  tsmc_Slforge14/1 -> tsmc_Slforge21/1
  tsmc_Slforge18/1 -> tsmc_Slforge4/1, tsmc_Slforge5/2
  tsmc_Slforge7/1 -> tsmc_Slforge18/1
  tsmc_Slforge1/1 -> tsmc_Slforge3/1
  tsmc_Slforge25/1 -> tsmc_Slforge17/2
  tsmc_Slforge8/2 -> tsmc_Slforge5/1
  tsmc_Slforge6/1 -> tsmc_Slforge21/2
  tsmc_Slforge4/1 -> tsmc_Slforge22/2
  tsmc_Slforge16/1 -> tsmc_Slforge15/1
  tsmc_Slforge3/1 -> tsmc_Slforge13/1
  tsmc_Slforge19/1 -> tsmc_Slforge20/2, tsmc_Slforge6/1
  tsmc_Slforge10/1 -> tsmc_Slforge14/1
  tsmc_Slforge22/1 -> tsmc_Slforge16/1
  tsmc_Slforge12/1 -> tsmc_Slforge14/2
  tsmc_Slforge9/1 -> tsmc_Slforge26/1
  tsmc_Slforge26/1 -> tsmc_Slforge20/1
  tsmc_Slforge17/1 -> tsmc_Slforge27/1
  tsmc_Slforge27/1 -> tsmc_Slforge22/1

== system dimensions_equivalent/tsmc_Slforge82 ==
  tsmc_Slforge1 : Inport
  tsmc_Slforge24 : Inport  Port=2
  Action Port : ActionPort  ActionPortLabel=if { }
  tsmc_Slforge10 : Product  Inputs=**
  tsmc_Slforge11 : Math  Operator=mod  SignedPower=on  SaturateOnIntegerOverflow=on
  tsmc_Slforge12 : Sqrt  SaturateOnIntegerOverflow=on
  tsmc_Slforge13 : Gain  Gain=[-481493748.840802]
  tsmc_Slforge14 : simulink/Math Operations/MinMax Running Resettable  Function=min  vinit=0.0
  tsmc_Slforge15 : Bias  Bias=[-828014900.881313]
  tsmc_Slforge16 : DotProduct  InputSameDT=on  OutDataTypeStr=Inherit: Inherit via internal rule
  tsmc_Slforge17 : ComplexToRealImag
  tsmc_Slforge18 : Gain  Gain=[-647598959.475434]
  tsmc_Slforge19 : UnaryMinus
  tsmc_Slforge20 : PermuteDimensions
  tsmc_Slforge21 : Trigonometry
  tsmc_Slforge22 : simulink/Math Operations/MinMax Running Resettable  Function=min  vinit=0.0
  tsmc_Slforge23 : Constant  Value=[-100635351.188928]  SampleTime=1
  tsmc_Slforge25 : Delay
  tsmc_Slforge26 : Delay
  tsmc_Slforge3 : simulink/Continuous/PID Controller (2DOF)  Controller=PID  TimeDomain=Discrete-time  SampleTime=-1  IntegratorMethod=Forward Euler  FilterMethod=Forward Euler  Form=Parallel  UseFilter=on  ControllerParametersSource=internal  P=1  I=1  D=0  N=100  b=1  c=1  InitialConditionSource=internal  InitialConditionForIntegrator=0  InitialConditionForFilter=0  ExternalReset=none  LimitOutput=off  UpperSaturationLimit=inf  LowerSaturationLimit=-inf  LinearizeAsGain=off  AntiWindupMode=none  Kb=1  TrackingMode=off  Kt=1  PParamMin=[]  PParamMax=[]  IParamMin=[]  IParamMax=[]  DParamMin=[]  DParamMax=[]  NParamMin=[]  NParamMax=[]  bParamMin=[]  bParamMax=[]  cParamMin=[]  cParamMax=[]  KbParamMin=[]  KbParamMax=[]  KtParamMin=[]  KtParamMax=[]  POutMin=[]  POutMax=[]  IOutMin=[]  IOutMax=[]  DOutMin=[]  DOutMax=[]  NOutMin=[]  NOutMax=[]  bOutMin=[]  bOutMax=[]  cOutMin=[]  cOutMax=[]  KbOutMin=[]  KbOutMax=[]  KtOutMin=[]  KtOutMax=[]  IntegratorOutMin=[]  IntegratorOutMax=[]  FilterOutMin=[]  FilterOutMax=[]  SumOutMin=[]  SumOutMax=[]  Sum1OutMin=[]  Sum1OutMax=[]  Sum2OutMin=[]  Sum2OutMax=[]  Sum3OutMin=[]  Sum3OutMax=[]  SumI1OutMin=[]  SumI1OutMax=[]  SumI2OutMin=[]  SumI2OutMax=[]  SumI3OutMin=[]  SumI3OutMax=[]  SumDOutMin=[]  SumDOutMax=[]  SaturationOutMin=[]  SaturationOutMax=[]  IntegratorContinuousStateAttributes=''  IntegratorStateMustResolveToSignalObject=off  IntegratorRTWStateStorageClass=Auto  FilterContinuousStateAttributes=''  FilterStateMustResolveToSignalObject=off  FilterRTWStateStorageClass=Auto  DifferentiatorICPrevScaledInput=0  DifferentiatorOutMin=[]  DifferentiatorOutMax=[]  FilterDiffOutCoefMin=[]  FilterDiffOutCoefMax=[]  SumDenOutMin=[]  SumDenOutMax=[]  SumNumOutMin=[]  SumNumOutMax=[]  ReciprocalOutMin=[]  ReciprocalOutMax=[]  DivideOutMin=[]  DivideOutMax=[]  TunerSelectOption=Transfer Function Based (PID Tuner App)
  tsmc_Slforge4 : Rounding
  tsmc_Slforge5 : Squeeze
  tsmc_Slforge6 : Trigonometry
  tsmc_Slforge7 : Bias  Bias=[-787005517.541563]
  tsmc_Slforge8 : ComplexToMagnitudeAngle
  tsmc_Slforge9 : Polyval  Coefs=[ +2.081618890e-019, -1.441693666e-014, +4.719686976e-010, -8.536869453e-006, +1.621573104e-001, -8.087801117e+001 ]
  tsmc_Slforge2 : Outport  VectorParamsAs1DForOutWhenUnconnected=off
  wires:
  tsmc_Slforge8/1 -> tsmc_Slforge22/1
  tsmc_Slforge7/1 -> tsmc_Slforge2/1
  tsmc_Slforge21/1 -> tsmc_Slforge17/1
  tsmc_Slforge6/1 -> tsmc_Slforge7/1
  tsmc_Slforge16/1 -> tsmc_Slforge20/1
  tsmc_Slforge20/1 -> tsmc_Slforge22/2
  tsmc_Slforge13/1 -> tsmc_Slforge10/1
  tsmc_Slforge17/1 -> tsmc_Slforge15/1
  tsmc_Slforge17/2 -> tsmc_Slforge14/1
  tsmc_Slforge23/1 -> tsmc_Slforge16/1
  tsmc_Slforge18/1 -> tsmc_Slforge19/1
  tsmc_Slforge14/1 -> tsmc_Slforge16/2
  tsmc_Slforge15/1 -> tsmc_Slforge10/2
  tsmc_Slforge8/2 -> tsmc_Slforge13/1
  tsmc_Slforge9/1 -> tsmc_Slforge4/1, tsmc_Slforge8/1
  tsmc_Slforge3/1 -> tsmc_Slforge12/1
  tsmc_Slforge5/1 -> tsmc_Slforge18/1
  tsmc_Slforge11/1 -> tsmc_Slforge9/1
  tsmc_Slforge4/1 -> tsmc_Slforge6/1, tsmc_Slforge5/1
  tsmc_Slforge24/1 -> tsmc_Slforge21/1
  tsmc_Slforge1/1 -> tsmc_Slforge11/2
  tsmc_Slforge10/1 -> tsmc_Slforge14/2
  tsmc_Slforge22/1 -> tsmc_Slforge3/2
  tsmc_Slforge19/1 -> tsmc_Slforge25/1
  tsmc_Slforge25/1 -> tsmc_Slforge11/1
  tsmc_Slforge12/1 -> tsmc_Slforge26/1
  tsmc_Slforge26/1 -> tsmc_Slforge3/1

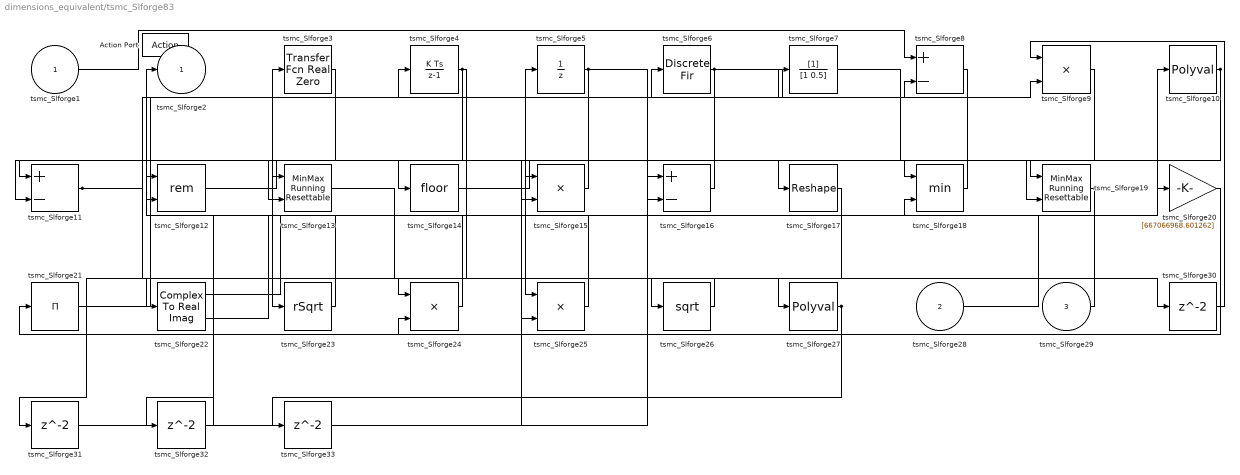
== system dimensions_equivalent/tsmc_Slforge83 ==
  tsmc_Slforge1 : Inport
  tsmc_Slforge28 : Inport  Port=2
  tsmc_Slforge29 : Inport  Port=3
  Action Port : ActionPort  ActionPortLabel=else { }
  tsmc_Slforge10 : Polyval  Coefs=[ +2.081618890e-019, -1.441693666e-014, +4.719686976e-010, -8.536869453e-006, +1.621573104e-001, -8.087801117e+001 ]
  tsmc_Slforge11 : Sum  Inputs=+-
  tsmc_Slforge12 : Math  Operator=rem  SignedPower=on  SaturateOnIntegerOverflow=on
  tsmc_Slforge13 : simulink/Math Operations/MinMax Running Resettable  Function=min  vinit=0.0
  tsmc_Slforge14 : Rounding
  tsmc_Slforge15 : Product  Inputs=**
  tsmc_Slforge16 : Sum  Inputs=+-
  tsmc_Slforge17 : Reshape
  tsmc_Slforge18 : MinMax  Inputs=2
  tsmc_Slforge19 : simulink/Math Operations/MinMax Running Resettable  Function=min  vinit=0.0
  tsmc_Slforge20 : Gain  Gain=[667066968.601262]
  tsmc_Slforge21 : Product  Inputs=*
  tsmc_Slforge22 : ComplexToRealImag
  tsmc_Slforge23 : Sqrt  Operator=rSqrt  AlgorithmType=Newton-Raphson  SaturateOnIntegerOverflow=on
  tsmc_Slforge24 : Product  Inputs=**
  tsmc_Slforge25 : Product
  tsmc_Slforge26 : Sqrt  SaturateOnIntegerOverflow=on
  tsmc_Slforge27 : Polyval  Coefs=[ +2.081618890e-019, -1.441693666e-014, +4.719686976e-010, -8.536869453e-006, +1.621573104e-001, -8.087801117e+001 ]
  tsmc_Slforge3 : simulink/Discrete/Transfer Fcn Real Zero  ZeroZ=0.75  ICPrevInput=0.0  DoSatur=off
      settings: SourceProductBaseCode=SL
  tsmc_Slforge{30..33} (4 alike) : Delay
  tsmc_Slforge4 : DiscreteIntegrator  SampleTime=-1  ICPrevOutput=DiscIntNeverNeededParam  ICPrevScaledInput=DiscIntNeverNeededParam
  tsmc_Slforge5 : UnitDelay  SampleTime=-1  HasFrameUpgradeWarning=on
  tsmc_Slforge6 : DiscreteFir
  tsmc_Slforge7 : DiscreteFilter
  tsmc_Slforge8 : Sum  Inputs=+-
  tsmc_Slforge9 : Product
  tsmc_Slforge2 : Outport  VectorParamsAs1DForOutWhenUnconnected=off
  wires:
  tsmc_Slforge15/1 -> tsmc_Slforge14/1
  tsmc_Slforge18/1 -> tsmc_Slforge6/1
  tsmc_Slforge1/1 -> tsmc_Slforge8/1
  tsmc_Slforge25/1 -> tsmc_Slforge2/1
  tsmc_Slforge17/1 -> tsmc_Slforge27/1
  tsmc_Slforge20/1 -> tsmc_Slforge21/1
  tsmc_Slforge3/1 -> tsmc_Slforge23/1
  tsmc_Slforge21/1 -> tsmc_Slforge8/2
  tsmc_Slforge24/1 -> tsmc_Slforge3/1
  tsmc_Slforge14/1 -> tsmc_Slforge17/1
  tsmc_Slforge16/1 -> tsmc_Slforge4/1
  tsmc_Slforge8/1 -> tsmc_Slforge18/1
  tsmc_Slforge28/1 -> tsmc_Slforge10/1
  tsmc_Slforge4/1 -> tsmc_Slforge24/1, tsmc_Slforge13/2
  tsmc_Slforge6/1 -> tsmc_Slforge9/2, tsmc_Slforge16/2
  tsmc_Slforge5/1 -> tsmc_Slforge20/1, tsmc_Slforge11/1, tsmc_Slforge11/2
  tsmc_Slforge12/1 -> tsmc_Slforge19/1
  tsmc_Slforge22/1 -> tsmc_Slforge18/2
  tsmc_Slforge10/1 -> tsmc_Slforge25/1, tsmc_Slforge25/2
  tsmc_Slforge23/1 -> tsmc_Slforge12/1
  tsmc_Slforge9/1 -> tsmc_Slforge13/1
  tsmc_Slforge11/1 -> tsmc_Slforge7/1, tsmc_Slforge26/1
  tsmc_Slforge19/1 -> tsmc_Slforge31/1, tsmc_Slforge32/1
  tsmc_Slforge29/1 -> tsmc_Slforge5/1
  tsmc_Slforge27/1 -> tsmc_Slforge24/2, tsmc_Slforge33/1
  tsmc_Slforge7/1 -> tsmc_Slforge19/2
  tsmc_Slforge26/1 -> tsmc_Slforge22/1
  tsmc_Slforge22/2 -> tsmc_Slforge15/1
  tsmc_Slforge13/1 -> tsmc_Slforge30/1
  tsmc_Slforge30/1 -> tsmc_Slforge9/1
  tsmc_Slforge31/1 -> tsmc_Slforge16/1
  tsmc_Slforge32/1 -> tsmc_Slforge12/2
  tsmc_Slforge33/1 -> tsmc_Slforge15/2

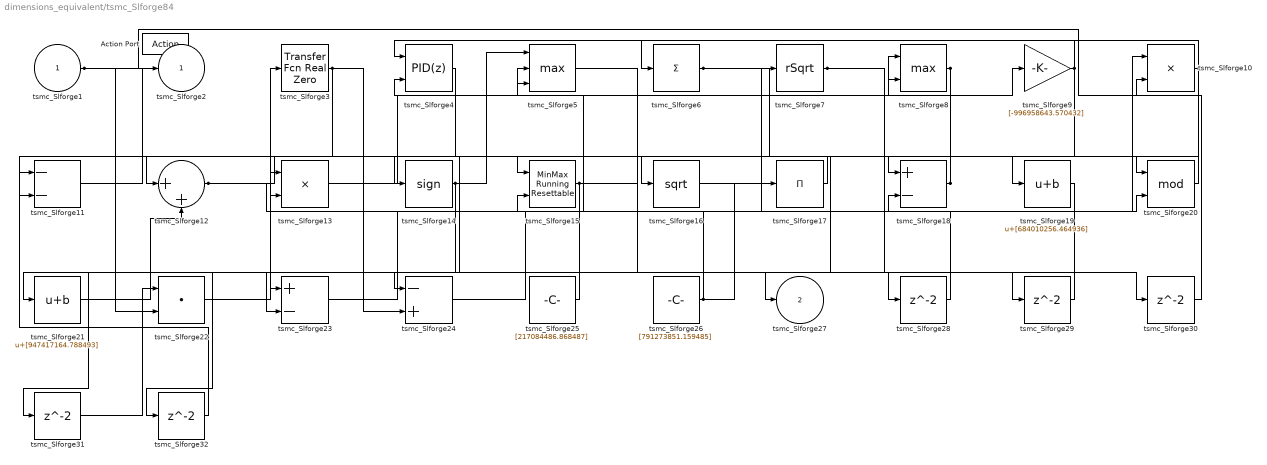
== system dimensions_equivalent/tsmc_Slforge84 ==
  tsmc_Slforge1 : Inport
  Action Port : ActionPort  ActionPortLabel=if { }
  tsmc_Slforge10 : Product
  tsmc_Slforge11 : Sum  Inputs=--
  tsmc_Slforge12 : Sum  Inputs=|++
  tsmc_Slforge13 : Product
  tsmc_Slforge14 : Signum
  tsmc_Slforge15 : simulink/Math Operations/MinMax Running Resettable  Function=min  vinit=0.0
  tsmc_Slforge16 : Sqrt  SaturateOnIntegerOverflow=on
  tsmc_Slforge17 : Product  Inputs=*
  tsmc_Slforge18 : Sum  Inputs=+-
  tsmc_Slforge19 : Bias  Bias=[684010256.464936]
  tsmc_Slforge20 : Math  Operator=mod  SignedPower=on  SaturateOnIntegerOverflow=on
  tsmc_Slforge21 : Bias  Bias=[947417164.788493]
  tsmc_Slforge22 : DotProduct  InputSameDT=on  OutDataTypeStr=Inherit: Inherit via internal rule
  tsmc_Slforge23 : Sum  Inputs=+-
  tsmc_Slforge24 : Sum  Inputs=-+
  tsmc_Slforge25 : Constant  Value=[217084486.868487]  SampleTime=1
  tsmc_Slforge26 : Constant  Value=[791273851.159485]  SampleTime=1
  tsmc_Slforge{28..32} (5 alike) : Delay
  tsmc_Slforge3 : simulink/Discrete/Transfer Fcn Real Zero  ZeroZ=0.75  ICPrevInput=0.0  DoSatur=off
      settings: SourceProductBaseCode=SL
  tsmc_Slforge4 : simulink/Continuous/PID Controller (2DOF)  Controller=PID  TimeDomain=Discrete-time  SampleTime=-1  IntegratorMethod=Forward Euler  FilterMethod=Forward Euler  Form=Parallel  UseFilter=on  ControllerParametersSource=internal  P=1  I=1  D=0  N=100  b=1  c=1  InitialConditionSource=internal  InitialConditionForIntegrator=0  InitialConditionForFilter=0  ExternalReset=none  LimitOutput=off  UpperSaturationLimit=inf  LowerSaturationLimit=-inf  LinearizeAsGain=off  AntiWindupMode=none  Kb=1  TrackingMode=off  Kt=1  PParamMin=[]  PParamMax=[]  IParamMin=[]  IParamMax=[]  DParamMin=[]  DParamMax=[]  NParamMin=[]  NParamMax=[]  bParamMin=[]  bParamMax=[]  cParamMin=[]  cParamMax=[]  KbParamMin=[]  KbParamMax=[]  KtParamMin=[]  KtParamMax=[]  POutMin=[]  POutMax=[]  IOutMin=[]  IOutMax=[]  DOutMin=[]  DOutMax=[]  NOutMin=[]  NOutMax=[]  bOutMin=[]  bOutMax=[]  cOutMin=[]  cOutMax=[]  KbOutMin=[]  KbOutMax=[]  KtOutMin=[]  KtOutMax=[]  IntegratorOutMin=[]  IntegratorOutMax=[]  FilterOutMin=[]  FilterOutMax=[]  SumOutMin=[]  SumOutMax=[]  Sum1OutMin=[]  Sum1OutMax=[]  Sum2OutMin=[]  Sum2OutMax=[]  Sum3OutMin=[]  Sum3OutMax=[]  SumI1OutMin=[]  SumI1OutMax=[]  SumI2OutMin=[]  SumI2OutMax=[]  SumI3OutMin=[]  SumI3OutMax=[]  SumDOutMin=[]  SumDOutMax=[]  SaturationOutMin=[]  SaturationOutMax=[]  IntegratorContinuousStateAttributes=''  IntegratorStateMustResolveToSignalObject=off  IntegratorRTWStateStorageClass=Auto  FilterContinuousStateAttributes=''  FilterStateMustResolveToSignalObject=off  FilterRTWStateStorageClass=Auto  DifferentiatorICPrevScaledInput=0  DifferentiatorOutMin=[]  DifferentiatorOutMax=[]  FilterDiffOutCoefMin=[]  FilterDiffOutCoefMax=[]  SumDenOutMin=[]  SumDenOutMax=[]  SumNumOutMin=[]  SumNumOutMax=[]  ReciprocalOutMin=[]  ReciprocalOutMax=[]  DivideOutMin=[]  DivideOutMax=[]  TunerSelectOption=Transfer Function Based (PID Tuner App)
  tsmc_Slforge5 : MinMax  Function=max  Inputs=3
  tsmc_Slforge6 : Sum  Inputs=+
  tsmc_Slforge7 : Sqrt  Operator=rSqrt  AlgorithmType=Newton-Raphson  SaturateOnIntegerOverflow=on
  tsmc_Slforge8 : MinMax  Function=max  Inputs=2
  tsmc_Slforge9 : Gain  Gain=[-996958643.570432]
  tsmc_Slforge2 : Outport  VectorParamsAs1DForOutWhenUnconnected=off
  tsmc_Slforge27 : Outport  Port=2  VectorParamsAs1DForOutWhenUnconnected=off
  wires:
  tsmc_Slforge26/1 -> tsmc_Slforge17/1, tsmc_Slforge5/2
  tsmc_Slforge12/1 -> tsmc_Slforge16/1, tsmc_Slforge15/2, tsmc_Slforge18/2
  tsmc_Slforge6/1 -> tsmc_Slforge20/1, tsmc_Slforge8/2
  tsmc_Slforge9/1 -> tsmc_Slforge19/1, tsmc_Slforge4/1
  tsmc_Slforge17/1 -> tsmc_Slforge12/1
  tsmc_Slforge22/1 -> tsmc_Slforge3/1
  tsmc_Slforge24/1 -> tsmc_Slforge7/1
  tsmc_Slforge20/1 -> tsmc_Slforge2/1
  tsmc_Slforge8/1 -> tsmc_Slforge27/1, tsmc_Slforge5/3
  tsmc_Slforge13/1 -> tsmc_Slforge8/1
  tsmc_Slforge21/1 -> tsmc_Slforge12/2
  tsmc_Slforge16/1 -> tsmc_Slforge20/2
  tsmc_Slforge7/1 -> tsmc_Slforge29/1, tsmc_Slforge30/1
  tsmc_Slforge14/1 -> tsmc_Slforge23/2, tsmc_Slforge5/1
  tsmc_Slforge18/1 -> tsmc_Slforge13/1, tsmc_Slforge4/2
  tsmc_Slforge15/1 -> tsmc_Slforge9/1, tsmc_Slforge31/1
  tsmc_Slforge4/1 -> tsmc_Slforge14/1
  tsmc_Slforge3/1 -> tsmc_Slforge11/2, tsmc_Slforge24/2
  tsmc_Slforge11/1 -> tsmc_Slforge15/1
  tsmc_Slforge1/1 -> tsmc_Slforge18/1, tsmc_Slforge22/2
  tsmc_Slforge25/1 -> tsmc_Slforge21/1
  tsmc_Slforge10/1 -> tsmc_Slforge6/1, tsmc_Slforge24/1
  tsmc_Slforge23/1 -> tsmc_Slforge10/1
  tsmc_Slforge5/1 -> tsmc_Slforge28/1
  tsmc_Slforge28/1 -> tsmc_Slforge13/2
  tsmc_Slforge29/1 -> tsmc_Slforge23/1
  tsmc_Slforge30/1 -> tsmc_Slforge10/2
  tsmc_Slforge31/1 -> tsmc_Slforge22/1
  tsmc_Slforge19/1 -> tsmc_Slforge32/1
  tsmc_Slforge32/1 -> tsmc_Slforge11/1

== system dimensions_equivalent/tsmc_Slforge85 ==
  tsmc_Slforge1 : Inport
  tsmc_Slforge21 : Inport  Port=2
  Action Port : ActionPort  ActionPortLabel=else { }
  tsmc_Slforge10 : simulink/Math Operations/MinMax Running Resettable  Function=min  vinit=0.0
  tsmc_Slforge11 : Math  Operator=hypot  SignedPower=on  SaturateOnIntegerOverflow=on
  tsmc_Slforge12 : ComplexToRealImag
  tsmc_Slforge13 : Sum  Inputs=|++
  tsmc_Slforge14 : Squeeze
  tsmc_Slforge15 : Gain  Gain=[-564250234.623791]
  tsmc_Slforge16 : Sum  Inputs=|++
  tsmc_Slforge17 : Sqrt  SaturateOnIntegerOverflow=on
  tsmc_Slforge18 : Constant  Value=[578256032.920959]  SampleTime=1
  tsmc_Slforge19 : Constant  Value=[589351854.681151]  SampleTime=1
  tsmc_Slforge20 : Constant  Value=[-120268038.215499]  SampleTime=1
  tsmc_Slforge3 : simulink/Math Operations/Slider Gain  gain=1  low=0  high=2
  tsmc_Slforge4 : Sqrt  Operator=rSqrt  AlgorithmType=Newton-Raphson  SaturateOnIntegerOverflow=on
  tsmc_Slforge5 : Product
  tsmc_Slforge6 : Sqrt  SaturateOnIntegerOverflow=on
  tsmc_Slforge7 : Bias  Bias=[-642271219.027506]
  tsmc_Slforge8 : Product  Inputs=**
  tsmc_Slforge9 : UnaryMinus
  tsmc_Slforge2 : Outport  VectorParamsAs1DForOutWhenUnconnected=off
  tsmc_Slforge22 : Outport  Port=2  VectorParamsAs1DForOutWhenUnconnected=off
  wires:
  tsmc_Slforge7/1 -> tsmc_Slforge14/1
  tsmc_Slforge21/1 -> tsmc_Slforge22/1, tsmc_Slforge12/1
  tsmc_Slforge3/1 -> tsmc_Slforge8/1
  tsmc_Slforge16/1 -> tsmc_Slforge6/1
  tsmc_Slforge8/1 -> tsmc_Slforge2/1
  tsmc_Slforge4/1 -> tsmc_Slforge9/1
  tsmc_Slforge13/1 -> tsmc_Slforge16/1
  tsmc_Slforge17/1 -> tsmc_Slforge15/1
  tsmc_Slforge15/1 -> tsmc_Slforge13/1
  tsmc_Slforge12/1 -> tsmc_Slforge4/1
  tsmc_Slforge10/1 -> tsmc_Slforge5/1
  tsmc_Slforge18/1 -> tsmc_Slforge8/2
  tsmc_Slforge5/1 -> tsmc_Slforge13/2
  tsmc_Slforge12/2 -> tsmc_Slforge16/2
  tsmc_Slforge6/1 -> tsmc_Slforge3/1
  tsmc_Slforge20/1 -> tsmc_Slforge17/1
  tsmc_Slforge14/1 -> tsmc_Slforge5/2
  tsmc_Slforge9/1 -> tsmc_Slforge10/1
  tsmc_Slforge1/1 -> tsmc_Slforge11/1
  tsmc_Slforge19/1 -> tsmc_Slforge11/2, tsmc_Slforge10/2
  tsmc_Slforge11/1 -> tsmc_Slforge7/1

== system dimensions_equivalent/tsmc_Slforge86 ==
  tsmc_Slforge1 : Inport
  tsmc_Slforge28 : Inport  Port=2
  Action Port : ActionPort  ActionPortLabel=if { }
  tsmc_Slforge{5,10,12,23} (4 alike) : Polyval  Coefs=[ +2.081618890e-019, -1.441693666e-014, +4.719686976e-010, -8.536869453e-006, +1.621573104e-001, -8.087801117e+001 ]
  tsmc_Slforge11 : Sum  Inputs=|++
  tsmc_Slforge13 : Sum  Inputs=+-
  tsmc_Slforge14 : Bias  Bias=[120399615.316605]
  tsmc_Slforge15 : Gain  Gain=[474347022.955851]
  tsmc_Slforge16 : Gain  Gain=[-954146156.000825]
  tsmc_Slforge17 : DotProduct  InputSameDT=on  OutDataTypeStr=Inherit: Inherit via internal rule
  tsmc_Slforge18 : Signum
  tsmc_Slforge19 : Math  Operator=10^u  SignedPower=on  SaturateOnIntegerOverflow=on
  tsmc_Slforge20 : Assignment  DiagnosticForDimensions=Warning  IndexOptions=Index vector (dialog)  Indices=1  OutputSizes=1
  tsmc_Slforge21 : simulink/Math Operations/MinMax Running Resettable  Function=min  vinit=0.0
  tsmc_Slforge22 : Sqrt  SaturateOnIntegerOverflow=on
  tsmc_Slforge24 : Constant  Value=[567522517.478324]  SampleTime=1
  tsmc_Slforge25 : Constant  Value=[761140370.882788]  SampleTime=1
  tsmc_Slforge26 : Constant  Value=[337327788.302214]  SampleTime=1
  tsmc_Slforge27 : Constant  Value=[924263129.805910]  SampleTime=1
  tsmc_Slforge3 : simulink/Discrete/Transfer Fcn Real Zero  ZeroZ=0.75  ICPrevInput=0.0  DoSatur=off
      settings: SourceProductBaseCode=SL
  tsmc_Slforge30 : Delay
  tsmc_Slforge4 : Reshape
  tsmc_Slforge6 : Sqrt  SaturateOnIntegerOverflow=on
  tsmc_Slforge7 : Rounding
  tsmc_Slforge8 : Sin  TimeSource=Use external signal  SampleTime=0
  tsmc_Slforge9 : ComplexToRealImag
  tsmc_Slforge2 : Outport  VectorParamsAs1DForOutWhenUnconnected=off
  tsmc_Slforge29 : Outport  Port=2  VectorParamsAs1DForOutWhenUnconnected=off
  wires:
  tsmc_Slforge25/1 -> tsmc_Slforge2/1
  tsmc_Slforge1/1 -> tsmc_Slforge6/1
  tsmc_Slforge19/1 -> tsmc_Slforge29/1
  tsmc_Slforge5/1 -> tsmc_Slforge9/1
  tsmc_Slforge17/1 -> tsmc_Slforge21/1
  tsmc_Slforge6/1 -> tsmc_Slforge13/1
  tsmc_Slforge14/1 -> tsmc_Slforge5/1
  tsmc_Slforge10/1 -> tsmc_Slforge21/2
  tsmc_Slforge15/1 -> tsmc_Slforge12/1
  tsmc_Slforge9/1 -> tsmc_Slforge22/1
  tsmc_Slforge8/1 -> tsmc_Slforge17/1
  tsmc_Slforge7/1 -> tsmc_Slforge4/1
  tsmc_Slforge4/1 -> tsmc_Slforge19/1
  tsmc_Slforge16/1 -> tsmc_Slforge18/1
  tsmc_Slforge28/1 -> tsmc_Slforge15/1
  tsmc_Slforge26/1 -> tsmc_Slforge16/1
  tsmc_Slforge13/1 -> tsmc_Slforge11/1
  tsmc_Slforge12/1 -> tsmc_Slforge17/2
  tsmc_Slforge27/1 -> tsmc_Slforge8/1
  tsmc_Slforge18/1 -> tsmc_Slforge11/2
  tsmc_Slforge3/1 -> tsmc_Slforge23/1
  tsmc_Slforge21/1 -> tsmc_Slforge14/1
  tsmc_Slforge20/1 -> tsmc_Slforge10/1
  tsmc_Slforge24/1 -> tsmc_Slforge13/2
  tsmc_Slforge9/2 -> tsmc_Slforge3/1
  tsmc_Slforge23/1 -> tsmc_Slforge7/1
  tsmc_Slforge11/1 -> tsmc_Slforge20/2
  tsmc_Slforge22/1 -> tsmc_Slforge30/1
  tsmc_Slforge30/1 -> tsmc_Slforge20/1

== system dimensions_equivalent/tsmc_Slforge87 ==
  tsmc_Slforge1 : Inport
  Action Port : ActionPort  ActionPortLabel=else { }
  tsmc_Slforge10 : Bias  Bias=[796354684.838629]
  tsmc_Slforge11 : ComplexToRealImag
  tsmc_Slforge12 : PermuteDimensions
  tsmc_Slforge13 : Sum  Inputs=|++
  tsmc_Slforge14 : Rounding
  tsmc_Slforge15 : Assignment  DiagnosticForDimensions=Warning  IndexOptions=Index vector (dialog)  Indices=1  OutputSizes=1
  tsmc_Slforge16 : simulink/Math Operations/MinMax Running Resettable  Function=min  vinit=0.0
  tsmc_Slforge17 : Sin  TimeSource=Use external signal  SampleTime=0
  tsmc_Slforge18 : simulink/Math Operations/Slider Gain  gain=1  low=0  high=2
  tsmc_Slforge19 : DotProduct  InputSameDT=on  OutDataTypeStr=Inherit: Inherit via internal rule
  tsmc_Slforge20 : Product  Inputs=**
  tsmc_Slforge21 : Math  Operator=conj  SignedPower=on  SaturateOnIntegerOverflow=on
  tsmc_Slforge22 : Constant  Value=[790544158.777945]  SampleTime=1
  tsmc_Slforge23 : Constant  Value=[751453744.434792]  SampleTime=1
  tsmc_Slforge25 : Delay
  tsmc_Slforge26 : Delay
  tsmc_Slforge27 : Delay
  tsmc_Slforge3 : DiscreteStateSpace  SampleTime=-1
  tsmc_Slforge4 : DiscreteFir
  tsmc_Slforge5 : Delay  ShowEnablePort=on
      settings: InputPortMap=u0,e6
  tsmc_Slforge6 : simulink/Math Operations/MinMax Running Resettable  Function=min  vinit=0.0
  tsmc_Slforge7 : Sum  Inputs=-+
  tsmc_Slforge8 : Product
  tsmc_Slforge9 : Sum  Inputs=+-
  tsmc_Slforge2 : Outport  VectorParamsAs1DForOutWhenUnconnected=off
  tsmc_Slforge24 : Outport  Port=2  VectorParamsAs1DForOutWhenUnconnected=off
  wires:
  tsmc_Slforge12/1 -> tsmc_Slforge18/1
  tsmc_Slforge23/1 -> tsmc_Slforge19/1
  tsmc_Slforge17/1 -> tsmc_Slforge8/1
  tsmc_Slforge10/1 -> tsmc_Slforge4/1, tsmc_Slforge14/1
  tsmc_Slforge20/1 -> tsmc_Slforge11/1
  tsmc_Slforge4/1 -> tsmc_Slforge17/1, tsmc_Slforge24/1
  tsmc_Slforge16/1 -> tsmc_Slforge8/2
  tsmc_Slforge15/1 -> tsmc_Slforge5/2, tsmc_Slforge26/1
  tsmc_Slforge11/1 -> tsmc_Slforge10/1
  tsmc_Slforge7/1 -> tsmc_Slforge2/1
  tsmc_Slforge18/1 -> tsmc_Slforge20/1, tsmc_Slforge15/2, tsmc_Slforge27/1
  tsmc_Slforge22/1 -> tsmc_Slforge19/2
  tsmc_Slforge5/1 -> tsmc_Slforge16/1, tsmc_Slforge7/2
  tsmc_Slforge11/2 -> tsmc_Slforge16/2
  tsmc_Slforge9/1 -> tsmc_Slforge15/1
  tsmc_Slforge1/1 -> tsmc_Slforge7/1
  tsmc_Slforge8/1 -> tsmc_Slforge6/1
  tsmc_Slforge19/1 -> tsmc_Slforge13/1
  tsmc_Slforge3/1 -> tsmc_Slforge6/2, tsmc_Slforge9/2, tsmc_Slforge13/2
  tsmc_Slforge21/1 -> tsmc_Slforge20/2
  tsmc_Slforge13/1 -> tsmc_Slforge21/1
  tsmc_Slforge14/1 -> tsmc_Slforge5/1
  tsmc_Slforge6/1 -> tsmc_Slforge25/1
  tsmc_Slforge25/1 -> tsmc_Slforge3/1
  tsmc_Slforge26/1 -> tsmc_Slforge9/1
  tsmc_Slforge27/1 -> tsmc_Slforge12/1
